simulink model "Logical_architecture"  (R2023b)
settings: Solver=VariableStepAuto  StartTime=0.0  StopTime=10.0  RelTol=1e-3
settings Model: Creator=Cristian  LastModifiedBy=Cristian

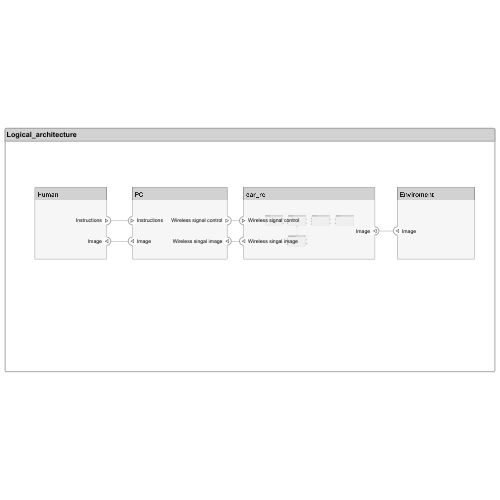
[thumbnail: Simulink's stored preview of the top-level diagram]
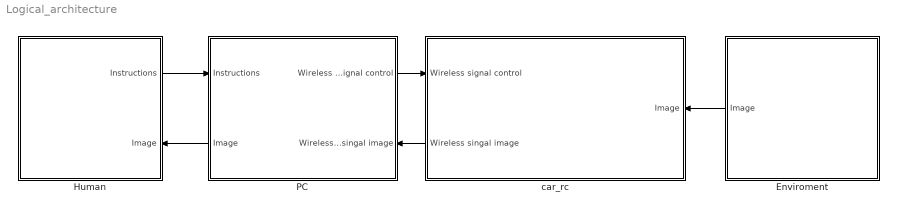
== system Logical_architecture ==
  Enviroment : Subsystem
      settings: PortSchema="{\"entries\":[{\"content\":{\"headerSize\":26,\"margin\":15,\"minimumSpacing\":25,\"sides\":[{\"content\":{\"connectorIds\":[\"Out1\"]},\"type\":\"ConnectorPlacement.EquallySpacedRectSide\",\"uuid\":\"a4c63610-ce53-4263-bc32-11f7e141828d\"},{\"content\":{\"side\":\"RIGHT\"},\"type\":\"ConnectorPlacement.EquallySpacedRectSide\",\"uuid\":\"7388023e-6661-4314-a5ba-fe6a68600945\"},{\"content\":{\"side\":\"TOP\"},\"type\":\"ConnectorPlacement.EquallySpacedRectSide\",\"uuid\":\"a8a6465a-b279-4272-9cd6-de33cf491c4f\"}]},\"type\":\"ConnectorPlacement.EquallySpacedConnector\",\"uuid\":\"83902977-a181-41b3-bc45-d69d98624d59\"}],\"packageUris\":[\"http://schema.mathworks.com/mf0/Connector/R2020b\"],\"version\":\"1.0\"}"
  Human : Subsystem
      settings: PortSchema="{\"entries\":[{\"content\":{\"headerSize\":26,\"margin\":15,\"minimumSpacing\":25,\"sides\":[{\"content\":{},\"type\":\"ConnectorPlacement.EquallySpacedRectSide\",\"uuid\":\"a4c63610-ce53-4263-bc32-11f7e141828d\"},{\"content\":{\"connectorIds\":[\"Out1\",\"In1\"],\"side\":\"RIGHT\"},\"type\":\"ConnectorPlacement.EquallySpacedRectSide\",\"uuid\":\"7388023e-6661-4314-a5ba-fe6a68600945\"},{\"content\":{\"side\":\"TOP\"},\"type\":\"ConnectorPlacement.EquallySpacedRectSide\",\"uuid\":\"a8a6465a-b279-4272-9cd6-de33cf491c4f\"}]},\"type\":\"ConnectorPlacement.EquallySpacedConnector\",\"uuid\":\"83902977-a181-41b3-bc45-d69d98624d59\"}],\"packageUris\":[\"http://schema.mathworks.com/mf0/Connector/R2020b\"],\"version\":\"1.0\"}"
  PC : Subsystem
      settings: PortSchema="{\"entries\":[{\"content\":{\"headerSize\":26,\"margin\":15,\"minimumSpacing\":25,\"sides\":[{\"content\":{\"connectorIds\":[\"In1\",\"Out1\"]},\"type\":\"ConnectorPlacement.EquallySpacedRectSide\",\"uuid\":\"a4c63610-ce53-4263-bc32-11f7e141828d\"},{\"content\":{\"connectorIds\":[\"Out2\",\"In2\"],\"side\":\"RIGHT\"},\"type\":\"ConnectorPlacement.EquallySpacedRectSide\",\"uuid\":\"7388023e-6661-4314-a5ba-fe6a68600945\"},{\"content\":{\"side\":\"TOP\"},\"type\":\"ConnectorPlacement.EquallySpacedRectSide\",\"uuid\":\"a8a6465a-b279-4272-9cd6-de33cf491c4f\"},{\"content\":{\"side\":\"BOTTOM\"},\"type\":\"ConnectorPlacement.EquallySpacedRectSide\",\"uuid\":\"8700fdea-8209-4825-9aa9-0f3498ee9306\"}]},\"type\":\"ConnectorPlacement.EquallySpacedConnector\",\"uuid\":\"83902977-a181-41b3-bc45-d69d98624d59\"}],\"packageUris\":[\"http://schema.mathworks.com/mf0/Connector/R2020b\"],\"version\":\"1.0\"}"
  car_rc : Subsystem
      settings: PortSchema="{\"entries\":[{\"content\":{\"headerSize\":26,\"margin\":15,\"minimumSpacing\":25,\"sides\":[{\"content\":{\"connectorIds\":[\"In2\",\"Out1\"]},\"type\":\"ConnectorPlacement.EquallySpacedRectSide\",\"uuid\":\"a4c63610-ce53-4263-bc32-11f7e141828d\"},{\"content\":{\"connectorIds\":[\"In1\"],\"side\":\"RIGHT\"},\"type\":\"ConnectorPlacement.EquallySpacedRectSide\",\"uuid\":\"7388023e-6661-4314-a5ba-fe6a68600945\"},{\"content\":{\"side\":\"TOP\"},\"type\":\"ConnectorPlacement.EquallySpacedRectSide\",\"uuid\":\"a8a6465a-b279-4272-9cd6-de33cf491c4f\"},{\"content\":{\"side\":\"BOTTOM\"},\"type\":\"ConnectorPlacement.EquallySpacedRectSide\",\"uuid\":\"d61feb0a-fa31-423e-9495-7042a628354c\"}]},\"type\":\"ConnectorPlacement.EquallySpacedConnector\",\"uuid\":\"83902977-a181-41b3-bc45-d69d98624d59\"}],\"packageUris\":[\"http://schema.mathworks.com/mf0/Connector/R2020b\"],\"version\":\"1.0\"}"
  wires:
  Enviroment/1(Image) -> car_rc/1(Image)
  PC/2(Wireless signal control) -> car_rc/2(Wireless signal control)
  car_rc/1(Wireless singal image) -> PC/2(Wireless singal image)
  Human/1(Instructions) -> PC/1(Instructions)
  PC/1(Image) -> Human/1(Image)

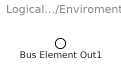
== system Logical_architecture/Enviroment ==
  Bus Element Out1 : Outport  PortName=Image

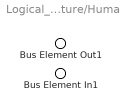
== system Logical_architecture/Human ==
  Bus Element In1 : Inport  PortName=Image
  Bus Element Out1 : Outport  PortName=Instructions

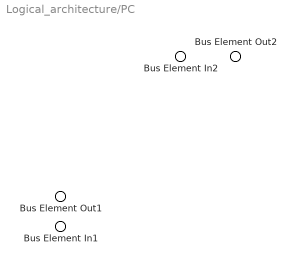
== system Logical_architecture/PC ==
  Bus Element In2 : Inport  PortName=Instructions
  Bus Element In1 : Inport  Port=2  PortName=Wireless singal image
  Bus Element Out2 : Outport  PortName=Image
  Bus Element Out1 : Outport  Port=2  PortName=Wireless signal control

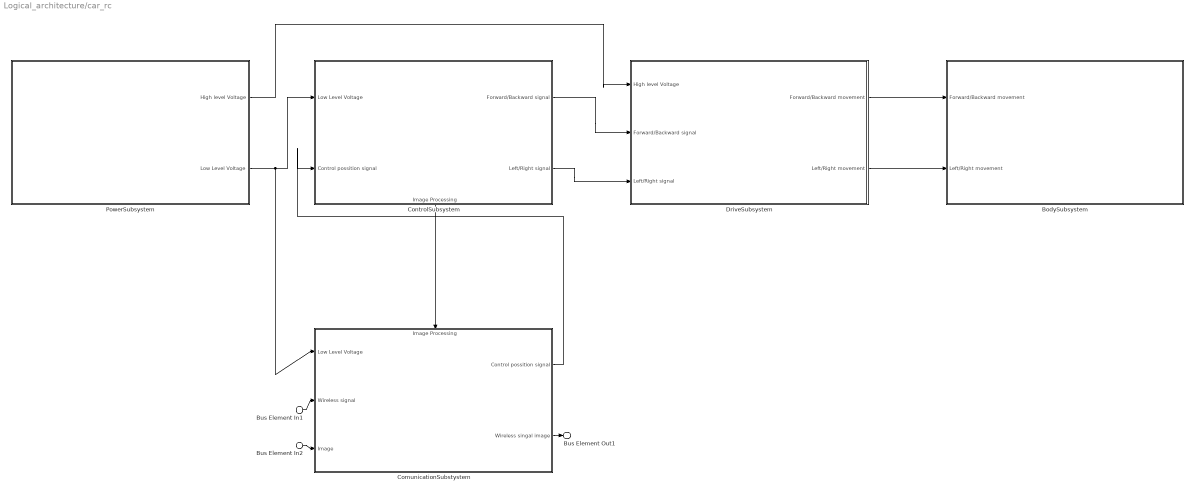
== system Logical_architecture/car_rc ==
  Bus Element In2 : Inport  PortName=Image
  Bus Element In1 : Inport  Port=2  PortName=Wireless signal control
  BodySubsystem : Subsystem
      settings: PortSchema="{\"entries\":[{\"content\":{\"headerSize\":26,\"margin\":15,\"minimumSpacing\":25,\"sides\":[{\"content\":{\"connectorIds\":[\"In1\",\"In2\"]},\"type\":\"ConnectorPlacement.EquallySpacedRectSide\",\"uuid\":\"a4c63610-ce53-4263-bc32-11f7e141828d\"},{\"content\":{\"side\":\"RIGHT\"},\"type\":\"ConnectorPlacement.EquallySpacedRectSide\",\"uuid\":\"7388023e-6661-4314-a5ba-fe6a68600945\"},{\"content\":{\"side\":\"TOP\"},\"type\":\"ConnectorPlacement.EquallySpacedRectSide\",\"uuid\":\"a8a6465a-b279-4272-9cd6-de33cf491c4f\"}]},\"type\":\"ConnectorPlacement.EquallySpacedConnector\",\"uuid\":\"83902977-a181-41b3-bc45-d69d98624d59\"}],\"packageUris\":[\"http://schema.mathworks.com/mf0/Connector/R2020b\"],\"version\":\"1.0\"}"
  ComunicationSubstystem : Subsystem
      settings: PortSchema="{\"entries\":[{\"content\":{\"headerSize\":26,\"margin\":15,\"minimumSpacing\":25,\"sides\":[{\"content\":{\"connectorIds\":[\"In2\",\"In3\",\"In4\"]},\"type\":\"ConnectorPlacement.EquallySpacedRectSide\",\"uuid\":\"a4c63610-ce53-4263-bc32-11f7e141828d\"},{\"content\":{\"connectorIds\":[\"Out1\",\"Out2\"],\"side\":\"RIGHT\"},\"type\":\"ConnectorPlacement.EquallySpacedRectSide\",\"uuid\":\"7388023e-6661-4314-a5ba-fe6a68600945\"},{\"content\":{\"connectorIds\":[\"In1\"],\"side\":\"TOP\"},\"type\":\"ConnectorPlacement.EquallySpacedRectSide\",\"uuid\":\"a8a6465a-b279-4272-9cd6-de33cf491c4f\"}]},\"type\":\"ConnectorPlacement.EquallySpacedConnector\",\"uuid\":\"83902977-a181-41b3-bc45-d69d98624d59\"}],\"packageUris\":[\"http://schema.mathworks.com/mf0/Connector/R2020b\"],\"version\":\"1.0\"}"
  ControlSubsystem : Subsystem
      settings: PortSchema="{\"entries\":[{\"content\":{\"headerSize\":26,\"margin\":15,\"minimumSpacing\":25,\"sides\":[{\"content\":{\"connectorIds\":[\"In1\",\"In2\"]},\"type\":\"ConnectorPlacement.EquallySpacedRectSide\",\"uuid\":\"a4c63610-ce53-4263-bc32-11f7e141828d\"},{\"content\":{\"connectorIds\":[\"Out2\",\"Out3\"],\"side\":\"RIGHT\"},\"type\":\"ConnectorPlacement.EquallySpacedRectSide\",\"uuid\":\"7388023e-6661-4314-a5ba-fe6a68600945\"},{\"content\":{\"side\":\"TOP\"},\"type\":\"ConnectorPlacement.EquallySpacedRectSide\",\"uuid\":\"a8a6465a-b279-4272-9cd6-de33cf491c4f\"},{\"content\":{\"connectorIds\":[\"Out1\"],\"side\":\"BOTTOM\"},\"type\":\"ConnectorPlacement.EquallySpacedRectSide\",\"uuid\":\"3bdcc6f8-6c71-4771-ba1a-6955a103437c\"}]},\"type\":\"ConnectorPlacement.EquallySpacedConnector\",\"uuid\":\"83902977-a181-41b3-bc45-d69d98624d59\"}],\"packageUris\":[\"http://schema.mathworks.com/mf0/Connector/R2020b\"],\"version\":\"1.0\"}"
  DriveSubsystem : Subsystem
      settings: PortSchema="{\"entries\":[{\"content\":{\"headerSize\":26,\"margin\":15,\"minimumSpacing\":25,\"sides\":[{\"content\":{\"connectorIds\":[\"In1\",\"In2\",\"In3\"]},\"type\":\"ConnectorPlacement.EquallySpacedRectSide\",\"uuid\":\"a4c63610-ce53-4263-bc32-11f7e141828d\"},{\"content\":{\"connectorIds\":[\"Out1\",\"Out2\"],\"side\":\"RIGHT\"},\"type\":\"ConnectorPlacement.EquallySpacedRectSide\",\"uuid\":\"7388023e-6661-4314-a5ba-fe6a68600945\"},{\"content\":{\"side\":\"TOP\"},\"type\":\"ConnectorPlacement.EquallySpacedRectSide\",\"uuid\":\"a8a6465a-b279-4272-9cd6-de33cf491c4f\"}]},\"type\":\"ConnectorPlacement.EquallySpacedConnector\",\"uuid\":\"83902977-a181-41b3-bc45-d69d98624d59\"}],\"packageUris\":[\"http://schema.mathworks.com/mf0/Connector/R2020b\"],\"version\":\"1.0\"}"
  PowerSubsystem : Subsystem
      settings: PortSchema="{\"entries\":[{\"content\":{\"headerSize\":26,\"margin\":15,\"minimumSpacing\":25,\"sides\":[{\"content\":{},\"type\":\"ConnectorPlacement.EquallySpacedRectSide\",\"uuid\":\"a4c63610-ce53-4263-bc32-11f7e141828d\"},{\"content\":{\"connectorIds\":[\"Out1\",\"Out2\"],\"side\":\"RIGHT\"},\"type\":\"ConnectorPlacement.EquallySpacedRectSide\",\"uuid\":\"7388023e-6661-4314-a5ba-fe6a68600945\"},{\"content\":{\"side\":\"TOP\"},\"type\":\"ConnectorPlacement.EquallySpacedRectSide\",\"uuid\":\"a8a6465a-b279-4272-9cd6-de33cf491c4f\"}]},\"type\":\"ConnectorPlacement.EquallySpacedConnector\",\"uuid\":\"83902977-a181-41b3-bc45-d69d98624d59\"}],\"packageUris\":[\"http://schema.mathworks.com/mf0/Connector/R2020b\"],\"version\":\"1.0\"}"
  Bus Element Out1 : Outport  PortName=Wireless singal image
  wires:
  PowerSubsystem/1(High level Voltage) -> DriveSubsystem/1(High level Voltage)
  PowerSubsystem/2(Low Level Voltage) -> ControlSubsystem/1(Low Level Voltage), ComunicationSubstystem/2(Low Level Voltage)
  ControlSubsystem/2(Forward/Backward signal) -> DriveSubsystem/2(Forward/Backward signal)
  ControlSubsystem/3(Left/Right signal) -> DriveSubsystem/3(Left/Right signal)
  DriveSubsystem/1(Forward/Backward movement) -> BodySubsystem/1(Forward/Backward movement)
  DriveSubsystem/2(Left/Right movement) -> BodySubsystem/2(Left/Right movement)
  Bus Element In1/1 -> ComunicationSubstystem/3(Wireless signal)
  ComunicationSubstystem/2(Wireless singal image) -> Bus Element Out1/1
  ComunicationSubstystem/1(Control possition signal) -> ControlSubsystem/2(Control possition signal)
  ControlSubsystem/1(Image Processing) -> ComunicationSubstystem/1(Image Processing)
  Bus Element In2/1 -> ComunicationSubstystem/4(Image)

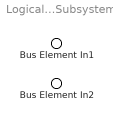
== system Logical_architecture/car_rc/BodySubsystem ==
  Bus Element In1 : Inport  PortName=Forward/Backward movement
  Bus Element In2 : Inport  Port=2  PortName=Left/Right movement

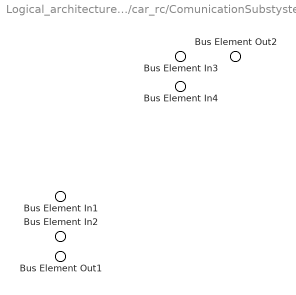
== system Logical_architecture/car_rc/ComunicationSubstystem ==
  Bus Element In4 : Inport  PortName=Image Processing
  Bus Element In1 : Inport  Port=2  PortName=Low Level Voltage
  Bus Element In3 : Inport  Port=3  PortName=Wireless signal
  Bus Element In2 : Inport  Port=4  PortName=Image
  Bus Element Out2 : Outport  PortName=Control possition signal
  Bus Element Out1 : Outport  Port=2  PortName=Wireless singal image

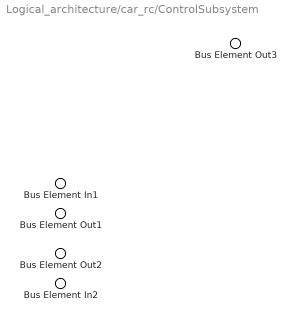
== system Logical_architecture/car_rc/ControlSubsystem ==
  Bus Element In1 : Inport  PortName=Low Level Voltage
  Bus Element In2 : Inport  Port=2  PortName=Control possition signal
  Bus Element Out3 : Outport  PortName=Image Processing
  Bus Element Out1 : Outport  Port=2  PortName=Forward/Backward signal
  Bus Element Out2 : Outport  Port=3  PortName=Left/Right signal

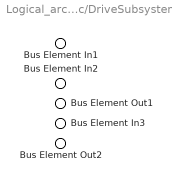
== system Logical_architecture/car_rc/DriveSubsystem ==
  Bus Element In1 : Inport  PortName=High level Voltage
  Bus Element In2 : Inport  Port=2  PortName=Forward/Backward signal
  Bus Element In3 : Inport  Port=3  PortName=Left/Right signal
  Bus Element Out1 : Outport  PortName=Forward/Backward movement
  Bus Element Out2 : Outport  Port=2  PortName=Left/Right movement

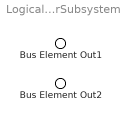
== system Logical_architecture/car_rc/PowerSubsystem ==
  Bus Element Out1 : Outport  PortName=High level Voltage
  Bus Element Out2 : Outport  Port=2  PortName=Low Level Voltage
